simulink model "fault_logic_model"  (R2025a)
settings: Solver=FixedStepDiscrete  StartTime=0.0  StopTime=20  FixedStep=1  RelTol=1e-3
libraries: simulink x2
settings Model: Creator=mahij  LastModifiedBy=mahij

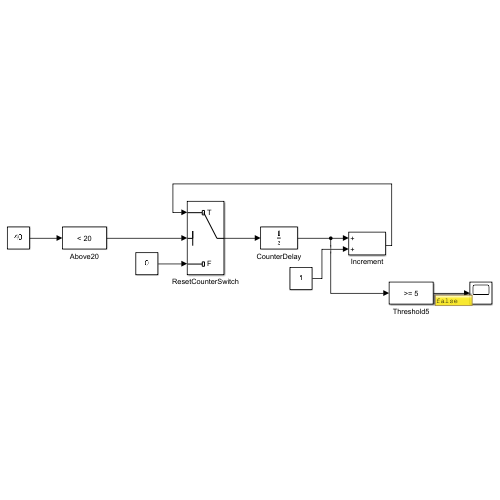
[thumbnail: Simulink's stored preview of the top-level diagram]
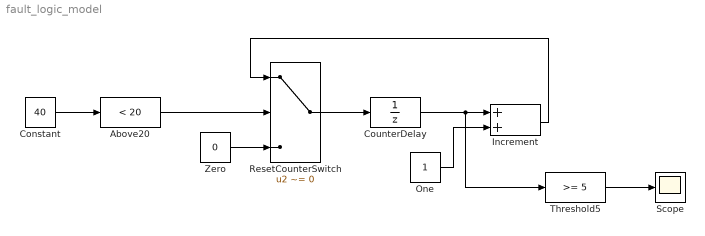
== system fault_logic_model ==
  Above20 : simulink/Logic and Bit Operations/Compare To Constant  relop=<  const=20  OutDataTypeStr=boolean
  Constant : Constant  Value=40
  CounterDelay : UnitDelay  HasFrameUpgradeWarning=on
  Increment : Sum
  One : Constant
  ResetCounterSwitch : Switch  Criteria=u2 ~= 0  Threshold=0.5  SaturateOnIntegerOverflow=off  InputSameDT=off
  Scope : Scope
  Threshold5 : simulink/Logic and Bit Operations/Compare To Constant  relop=>=  const=5  OutDataTypeStr=boolean
  Zero : Constant  Value=0
  wires:
  Constant/1 -> Above20/1
  Above20/1 -> ResetCounterSwitch/2
  Zero/1 -> ResetCounterSwitch/3
  Increment/1 -> ResetCounterSwitch/1
  ResetCounterSwitch/1 -> CounterDelay/1
  CounterDelay/1 -> Threshold5/1, Increment/1
  One/1 -> Increment/2
  Threshold5/1 -> Scope/1
